simulink model "Itc"  (Simulink 8.4)
settings: Solver=ode45  StartTime=0.0  StopTime=10.0  RelTol=1e-3
undefined symbols (not defined in the file): Itc_flgInjCutoffMan, Itc_flgInjTimeOverride, Itc_pManiFiltMax, Itc_rpmEngSpdHyst, Itc_rpmEngSpdMax, Itc_tiInjMan, Itc_tiInjMin, Itc_tiInjOffsetMan
settings Model: Creator=YAL9FE  LastModifiedBy=ric9fe
settings DebuggingCC: FcnCallInpInsideContextMsg=EnableAllAsWarning

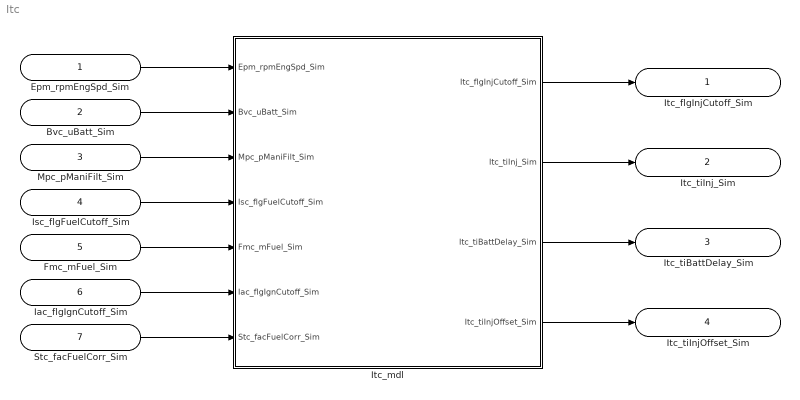
== system Itc ==
  Epm_rpmEngSpd_Sim : Inport
  Bvc_uBatt_Sim : Inport  Port=2
  Mpc_pManiFilt_Sim : Inport  Port=3
  Isc_flgFuelCutoff_Sim : Inport  Port=4
  Fmc_mFuel_Sim : Inport  Port=5
  Iac_flgIgnCutoff_Sim : Inport  Port=6
  Stc_facFuelCorr_Sim : Inport  Port=7
  Itc_mdl : Subsystem  mask(Functions){}
      mask help: InjectionTime
      mask Display:
      | image(imread('InjectionTime.jpg'))
      | port_label('input',1,'Epm_rpmEngSpd_Sim')
      | port_label('input',2,'Bvc_uBatt_Sim')
      | port_label('input',3,'Mpc_pManiFilt_Sim')
      | port_label('input',4,'Isc_flgFuelCutoff_Sim')
      | port_label('input',5,'Fmc_mFuel_Sim')
      | port_label('input',6,'Iac_flgIgnCutoff_Sim')
      | port_label('input',7,'Stc_facFuelCorr_Sim')
      | port_label('output',1,'Itc_flgInjCutoff_Sim')
      | port_label('output',2,'Itc_tiInj_Sim')
      | port_label('output',3,'Itc_tiBattDelay_Sim')
      | port_label('output',4,'Itc_tiInjOffset_Sim')
  Itc_flgInjCutoff_Sim : Outport
  Itc_tiInj_Sim : Outport  Port=2
  Itc_tiBattDelay_Sim : Outport  Port=3
  Itc_tiInjOffset_Sim : Outport  Port=4
  wires:
  Epm_rpmEngSpd_Sim/1 -> Itc_mdl/1(Epm_rpmEngSpd_Sim)
  Bvc_uBatt_Sim/1 -> Itc_mdl/2(Bvc_uBatt_Sim)
  Mpc_pManiFilt_Sim/1 -> Itc_mdl/3(Mpc_pManiFilt_Sim)
  Isc_flgFuelCutoff_Sim/1 -> Itc_mdl/4(Isc_flgFuelCutoff_Sim)
  Fmc_mFuel_Sim/1 -> Itc_mdl/5(Fmc_mFuel_Sim)
  Iac_flgIgnCutoff_Sim/1 -> Itc_mdl/6(Iac_flgIgnCutoff_Sim)
  Stc_facFuelCorr_Sim/1 -> Itc_mdl/7(Stc_facFuelCorr_Sim)
  Itc_mdl/1(Itc_flgInjCutoff_Sim) -> Itc_flgInjCutoff_Sim/1
  Itc_mdl/2(Itc_tiInj_Sim) -> Itc_tiInj_Sim/1
  Itc_mdl/3(Itc_tiBattDelay_Sim) -> Itc_tiBattDelay_Sim/1
  Itc_mdl/4(Itc_tiInjOffset_Sim) -> Itc_tiInjOffset_Sim/1

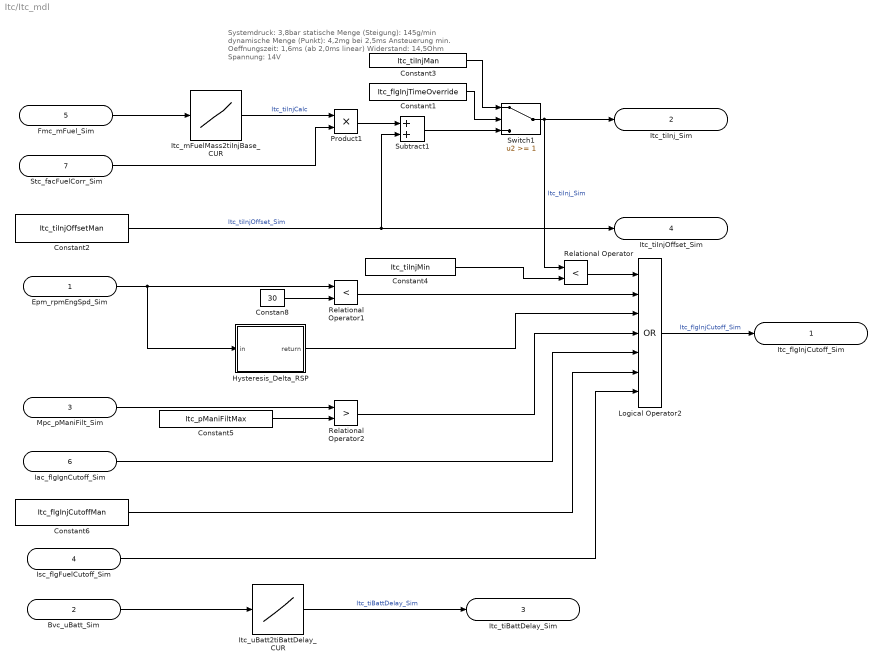
== system Itc/Itc_mdl ==
  note: Systemdruck:                                                                3,8bar
      | statische Menge (Steigung):                                      145g/min
      | dynamische Menge (Punkt):     4,2mg bei 2,5ms Ansteuerung
      | min. Oeffnungszeit:                              1,6ms (ab 2,0ms linear)
      | Widerstand:                                                                14,5Ohm
      | Spannung:                                                                         14V
  Epm_rpmEngSpd_Sim : Inport
  Bvc_uBatt_Sim : Inport  Port=2
  Mpc_pManiFilt_Sim : Inport  Port=3
  Isc_flgFuelCutoff_Sim : Inport  Port=4
  Fmc_mFuel_Sim : Inport  Port=5
  Iac_flgIgnCutoff_Sim : Inport  Port=6
  Stc_facFuelCorr_Sim : Inport  Port=7
  Constan8 : Constant  Value=30  OutDataTypeStr=single
  Constant1 : Constant  Value=Itc_flgInjTimeOverride
  Constant2 : Constant  Value=Itc_tiInjOffsetMan
  Constant3 : Constant  Value=Itc_tiInjMan
  Constant4 : Constant  Value=Itc_tiInjMin
  Constant5 : Constant  Value=Itc_pManiFiltMax
  Constant6 : Constant  Value=Itc_flgInjCutoffMan
  Hysteresis_Delta_RSP : Subsystem
      mask help: Hysteresis_Delta_RSP
      mask Display: image(imread('HysteresDeltaR.jpg'))
  Itc_mFuelMass2tiInjBase_CUR : Lookup_n-D  NumberOfTableDimensions=1  BreakpointsForDimension1=[1:3]  Table=[10 18 23]  ExtrapMethod=Clip  InputSameDT=on
  Itc_uBatt2tiBattDelay_CUR : Lookup_n-D  NumberOfTableDimensions=1  BreakpointsForDimension1=[1:3]  Table=[16 19 20]  ExtrapMethod=Clip  InputSameDT=on
  Logical Operator2 : Logic  Operator=OR  Inputs=7  AllPortsSameDT=off  OutDataTypeStr=boolean
  Product1 : Product  OutDataTypeStr=Inherit: Same as first input
  Relational Operator : RelationalOperator  Operator=<  OutDataTypeStr=boolean
  Relational Operator1 : RelationalOperator  Operator=<  OutDataTypeStr=boolean
  Relational Operator2 : RelationalOperator  Operator=>  OutDataTypeStr=boolean
  Subtract1 : Sum  OutDataTypeStr=Inherit: Same as first input
  Switch1 : Switch  Threshold=1
  Itc_flgInjCutoff_Sim : Outport
  Itc_tiInj_Sim : Outport  Port=2
  Itc_tiBattDelay_Sim : Outport  Port=3
  Itc_tiInjOffset_Sim : Outport  Port=4
  wires:
  Constant1/1 -> Switch1/2
  Constant3/1 -> Switch1/1
  Fmc_mFuel_Sim/1 -> Itc_mFuelMass2tiInjBase_CUR/1
  Itc_mFuelMass2tiInjBase_CUR/1 -> Product1/1  "Itc_tiInjCalc"
  Stc_facFuelCorr_Sim/1 -> Product1/2
  Product1/1 -> Subtract1/1
  Constant2/1 -> Subtract1/2, Itc_tiInjOffset_Sim/1  "Itc_tiInjOffset_Sim"
  Subtract1/1 -> Switch1/3
  Constant4/1 -> Relational Operator/2
  Switch1/1 -> Relational Operator/1, Itc_tiInj_Sim/1  "Itc_tiInj_Sim"
  Relational Operator/1 -> Logical Operator2/1
  Logical Operator2/1 -> Itc_flgInjCutoff_Sim/1  "Itc_flgInjCutoff_Sim"
  Epm_rpmEngSpd_Sim/1 -> Relational Operator1/1, Hysteresis_Delta_RSP/1(in)
  Constan8/1 -> Relational Operator1/2
  Relational Operator1/1 -> Logical Operator2/2
  Hysteresis_Delta_RSP/1(return) -> Logical Operator2/3
  Mpc_pManiFilt_Sim/1 -> Relational Operator2/1
  Constant5/1 -> Relational Operator2/2
  Relational Operator2/1 -> Logical Operator2/4
  Iac_flgIgnCutoff_Sim/1 -> Logical Operator2/5
  Constant6/1 -> Logical Operator2/6
  Isc_flgFuelCutoff_Sim/1 -> Logical Operator2/7
  Bvc_uBatt_Sim/1 -> Itc_uBatt2tiBattDelay_CUR/1
  Itc_uBatt2tiBattDelay_CUR/1 -> Itc_tiBattDelay_Sim/1  "Itc_tiBattDelay_Sim"

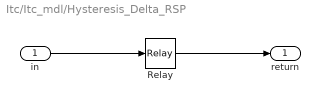
== system Itc/Itc_mdl/Hysteresis_Delta_RSP ==
  in : Inport
  Relay : Relay  OnSwitchValue=Itc_rpmEngSpdMax  OffSwitchValue=Itc_rpmEngSpdMax-Itc_rpmEngSpdHyst  OutDataTypeStr=Inherit: Inherit via back propagation
  return : Outport
  wires:
  Relay/1 -> return/1
  in/1 -> Relay/1
